simulink model "quadrotor_control_template"  (R2021a)
settings: Solver=VariableStepAuto  StartTime=0.0  StopTime=5  MaxStep=0.001  RelTol=1e-6
PreLoadFcn:
  | % first load parameters
  | initializeQuadrotorModel;
undefined symbols (not defined in the file): quadrotor, simPar
libraries: sharedtransform x1
settings Model: Creator=beniamino  LastModifiedBy=beniamino
settings SolverCC: AlgebraicLoopSolver=TrustRegion

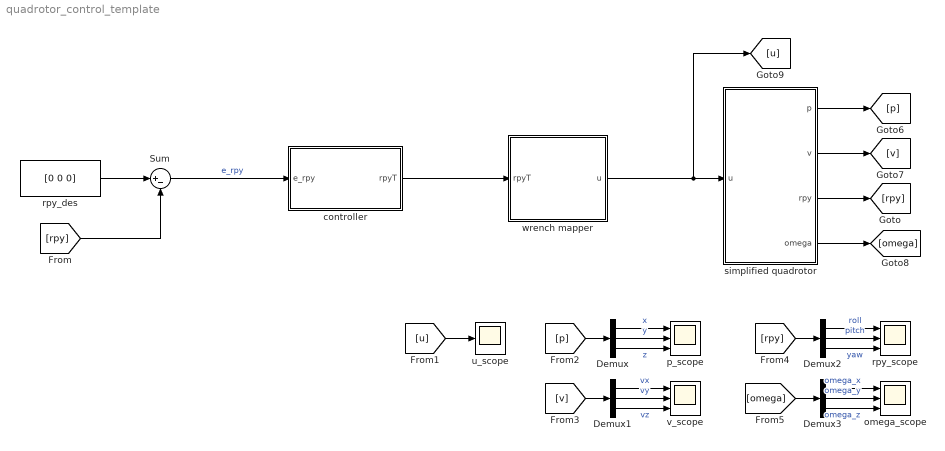
== system quadrotor_control_template ==
  Demux{,1..3} (4 alike) : Demux  Outputs=3
  Sum : Sum  Inputs=|+-
  controller : Subsystem
  omega_scope : Scope  NumInputPorts=3
  p_scope : Scope  NumInputPorts=3
  rpy_des : Constant  Value=[0 0 0]
  rpy_scope : Scope  NumInputPorts=3
  simplified quadrotor : Subsystem  mask(quadrotor model){F=quadrotor.mixer.F, M=quadrotor.mixer.M, mass=quadrotor.geometry.mass, gravity=simPar.g, inertia=quadrotor.geometry.I, maxRotorSpeed2=quadrotor.rotor.maxRotVelocity.^2, minRotorSpeed2=0, v_0=[0 0 0], omega_0=[0 0 0], ang_0=[0 0 0], p_0=[0 0 0]}
      mask prompts: F "F matrix"; M "M matrix"; mass "quadrotor mass"; inertia "inertia matrix"; maxRotorSpeed2 "Rotor max speed square"; minRotorSpeed2 "Rotor min speed square"; v_0 "initial linear velocity"; omega_0 "initial angular velocity"; ang_0 "initial angle"; p_0 "initial position"
      mask help: small angle simplified quadrotor model
      mask TypeOptions F: u2F/Gain
      mask TypeOptions M: u2M/Gain
      mask TypeOptions mass: mass/Value
      mask TypeOptions gravity: small angles rigid body dynamics/gravity/Value
      mask TypeOptions inertia: inertia/Value
      mask TypeOptions maxRotorSpeed2: saturate input/UpperLimit
      mask TypeOptions minRotorSpeed2: saturate input/LowerLimit
      mask TypeOptions v_0: small angles rigid body dynamics/ddp2dp/InitialCondition
      mask TypeOptions omega_0: small angles rigid body dynamics/domega2omega/InitialCondition
      mask TypeOptions ang_0: small angles rigid body dynamics/omega2ang/InitialCondition
      mask TypeOptions p_0: small angles rigid body dynamics/dp2p/InitialCondition
      mask DialogControl InitialConditionsGroupVar Prompt: Initial conditions
  u_scope : Scope
  v_scope : Scope  NumInputPorts=3
  wrench mapper : Subsystem  mask(wrench mapper){mapperMatrix=quadrotor.mixer.wrenchMapper}
      mask prompts: mapperMatrix "mapper matrix"
      mask help:
      | maps desired roll, pitch, yaw torque and total common thrust into the input vector u for a quadrotor.
      | input: [tau_roll, tau_pitch, tau_yaw, thrust]
      | input unit: [Nm, Nm, Nm, N]
      | output [u_1, u_2, u_3, u_3]
      | output unit: [rad^2/s^2]
      mask TypeOptions mapperMatrix: mapper/Gain
  wires:
  wrench mapper/1(u) -> [u], simplified quadrotor/1(u)
  simplified quadrotor/3(rpy) -> [rpy]
  simplified quadrotor/1(p) -> [p]
  simplified quadrotor/2(v) -> [v]
  simplified quadrotor/4(omega) -> [omega]
  rpy_des/1 -> Sum/1
  [rpy] -> Sum/2
  [u] -> u_scope/1
  Sum/1 -> controller/1(e_rpy)  "e_rpy"
  controller/1(rpyT) -> wrench mapper/1(rpyT)
  [p] -> Demux/1
  Demux/1 -> p_scope/1  "x"
  Demux/2 -> p_scope/2  "y"
  Demux/3 -> p_scope/3  "z"
  [v] -> Demux1/1
  Demux1/2 -> v_scope/2  "vy"
  Demux1/3 -> v_scope/3  "vz"
  Demux1/1 -> v_scope/1  "vx"
  [rpy] -> Demux2/1
  Demux2/2 -> rpy_scope/2  "pitch"
  Demux2/3 -> rpy_scope/3  "yaw"
  Demux2/1 -> rpy_scope/1  "roll"
  [omega] -> Demux3/1
  Demux3/2 -> omega_scope/2  "omega_y"
  Demux3/3 -> omega_scope/3  "omega_z"
  Demux3/1 -> omega_scope/1  "omega_x"

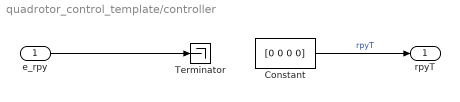
== system quadrotor_control_template/controller ==
  e_rpy : Inport
  Constant : Constant  Value=[0 0 0 0]
  Terminator : Terminator
  rpyT : Outport
  wires:
  e_rpy/1 -> Terminator/1
  Constant/1 -> rpyT/1  "rpyT"

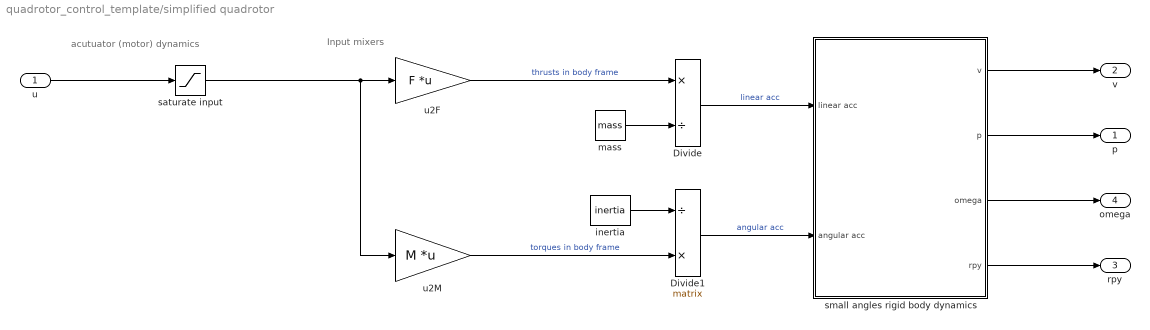
== system quadrotor_control_template/simplified quadrotor ==
  note: Input mixers
  note: acutuator (motor) dynamics
  u : Inport
  Divide : Product  Inputs=*/
  Divide1 : Product  Inputs=/*  Multiplication=Matrix(*)
  inertia : Constant  Value=inertia
  mass : Constant  Value=mass
  saturate input : Saturate  UpperLimit=maxRotorSpeed2  LowerLimit=minRotorSpeed2
  small angles rigid body dynamics : Subsystem
  u2F : Gain  Gain=F  Multiplication=Matrix(K*u)
  u2M : Gain  Gain=M  Multiplication=Matrix(K*u)
  p : Outport  PortDimensions=3
  v : Outport  Port=2  PortDimensions=3
  rpy : Outport  Port=3  PortDimensions=3
  omega : Outport  Port=4  PortDimensions=3
  wires:
  small angles rigid body dynamics/4(rpy) -> rpy/1
  small angles rigid body dynamics/3(omega) -> omega/1
  small angles rigid body dynamics/2(p) -> p/1
  small angles rigid body dynamics/1(v) -> v/1
  Divide1/1 -> small angles rigid body dynamics/2(angular acc)  "angular acc"
  Divide/1 -> small angles rigid body dynamics/1(linear acc)  "linear acc"
  u/1 -> saturate input/1
  inertia/1 -> Divide1/1
  u2M/1 -> Divide1/2  "torques in body frame"
  u2F/1 -> Divide/1  "thrusts in body frame"
  mass/1 -> Divide/2
  saturate input/1 -> u2F/1, u2M/1

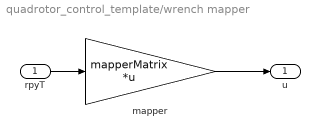
== system quadrotor_control_template/wrench mapper ==
  rpyT : Inport
  mapper : Gain  Gain=mapperMatrix  Multiplication=Matrix(K*u)
  u : Outport
  wires:
  mapper/1 -> u/1
  rpyT/1 -> mapper/1

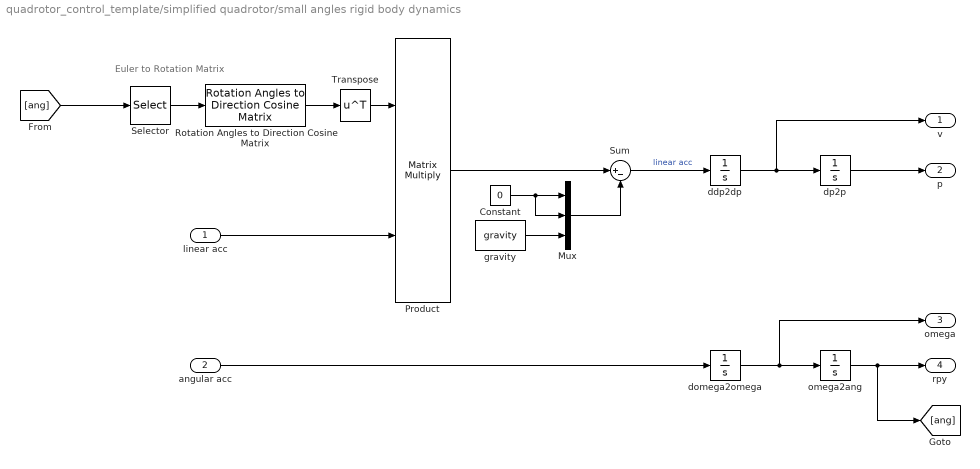
== system quadrotor_control_template/simplified quadrotor/small angles rigid body dynamics ==
  note: Euler to Rotation Matrix
  linear acc : Inport
  angular acc : Inport  Port=2
  Constant : Constant  Value=0
  Mux : Mux  Inputs=3
  Product : Product  Multiplication=Matrix(*)
  Rotation Angles to Direction Cosine Matrix : sharedtransform/Rotation Angles to Direction Cosine Matrix  rotationOrder=ZYX  aMode=aMode
      settings: SourceProductBaseCode=AE,PW,DR,MT,UV,VE
  Selector : Selector  InputPortWidth=3  IndexOptions=Index vector (dialog)  Indices=[3 2 1]  OutputSizes=1
  Sum : Sum  Inputs=|+-
  Transpose : Math  Operator=transpose  SaturateOnIntegerOverflow=on
  ddp2dp : Integrator  InitialCondition=v_0  ContinuousStateAttributes='v'
  domega2omega : Integrator  InitialCondition=omega_0  ContinuousStateAttributes='omega'
  dp2p : Integrator  InitialCondition=p_0  ContinuousStateAttributes='position'
  gravity : Constant  Value=gravity
  omega2ang : Integrator  InitialCondition=ang_0  ContinuousStateAttributes='rpy'
  v : Outport
  p : Outport  Port=2
  omega : Outport  Port=3
  rpy : Outport  Port=4
  wires:
  Mux/1 -> Sum/2
  [ang] -> Selector/1
  angular acc/1 -> domega2omega/1
  gravity/1 -> Mux/3
  ddp2dp/1 -> dp2p/1, v/1
  linear acc/1 -> Product/2
  Transpose/1 -> Product/1
  Product/1 -> Sum/1
  domega2omega/1 -> omega2ang/1, omega/1
  dp2p/1 -> p/1
  Sum/1 -> ddp2dp/1  "linear acc"
  Constant/1 -> Mux/1, Mux/2
  Selector/1 -> Rotation Angles to Direction Cosine Matrix/1
  omega2ang/1 -> [ang], rpy/1
  Rotation Angles to Direction Cosine Matrix/1 -> Transpose/1
